simulink model "derivador_purot_digital"  (Simulink 10.0)
settings: Solver=VariableStepAuto  StartTime=0.0  StopTime=2  RelTol=1e-3
settings Model: Creator=fernandopassold  LastModifiedBy=fernandopassold
settings DataIOCC: SaveFormat=Dataset
settings OptimizationCC: LifeSpan=auto
settings DebuggingCC: UnderspecifiedInitializationDetection=Simplified  MergeDetectMultiDrivingBlocksExec=error  SFUnexpectedBacktrackingDiag=error  SFNoUnconditionalDefaultTransitionDiag=error  SFExecutionAtInitializationDiag=warning
settings HardwareCC: ProdBitPerPointer=64  ProdBitPerSizeT=64  ProdBitPerPtrDiffT=64  ProdLargestAtomicFloat=Float  ProdIntDivRoundTo=Zero  ProdEndianess=LittleEndian  ProdWordSize=64  ProdHWDeviceType=Intel->x86-64 (Windows64)
settings ModelReferenceCC: PropagateSignalLabelsOutOfModel=on
settings CodeAppCC: StateflowObjectComments=off
settings GRTTargetCC: TargetLangStandard=C99 (ISO)  CombineOutputUpdateFcns=on  GRTInterface=off
settings ConfigComp: CovMetricSettings=dwe  CovHtmlReporting=off  CovSaveCumulativeToWorkspaceVar=off  CovSaveSingleToWorkspaceVar=off

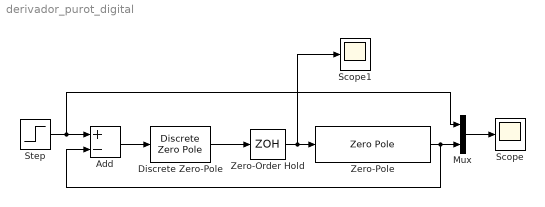
== system derivador_purot_digital ==
  Add : Sum  Inputs=+-
  Discrete Zero-Pole : DiscreteZeroPole  Poles=[0]  Gain=1  SampleTime=0.1
  Mux : Mux  Inputs=2
  Scope : Scope
  Scope1 : Scope
  Step : Step  SampleTime=0
  Zero-Order Hold : ZeroOrderHold  SampleTime=0.1
  Zero-Pole : ZeroPole  Zeros=[ ]  Poles=[-1 -2 -10]
  wires:
  Step/1 -> Mux/1, Add/1
  Mux/1 -> Scope/1
  Zero-Pole/1 -> Add/2, Mux/2
  Discrete Zero-Pole/1 -> Zero-Order Hold/1
  Zero-Order Hold/1 -> Scope1/1, Zero-Pole/1
  Add/1 -> Discrete Zero-Pole/1
